simulink model "Ejercicio_2"  (R2020a)
settings: Solver=ode3  StartTime=0.0  StopTime=100.0  FixedStep=0.01  RelTol=1e-3
undefined symbols (not defined in the file or in its folder): DiscIntNeverNeededParam
libraries: simulink x1
settings Model: EnablePacing=on  Creator=atien  LastModifiedBy=atien

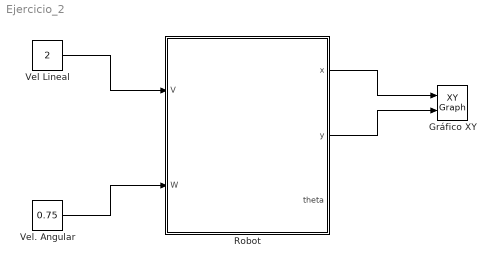
== system Ejercicio_2 ==
  Gráfico XY : simulink/Sinks/XY Graph  xmin=-10  xmax=10  ymin=-10  ymax=10  st=-1
  Robot : Subsystem
  Vel Lineal : Constant  Value=2
  Vel. Angular : Constant  Value=0.75
  wires:
  Vel Lineal/1 -> Robot/1(V)
  Robot/1(x) -> Gráfico XY/1
  Robot/2(y) -> Gráfico XY/2
  Vel. Angular/1 -> Robot/2(W)

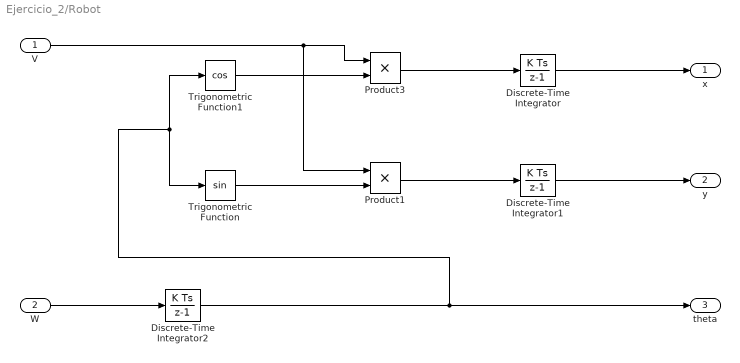
== system Ejercicio_2/Robot ==
  V : Inport
  W : Inport  Port=2
  Discrete-Time Integrator : DiscreteIntegrator  InitialCondition=-4  SampleTime=-1  ICPrevOutput=DiscIntNeverNeededParam  ICPrevScaledInput=DiscIntNeverNeededParam
  Discrete-Time Integrator1 : DiscreteIntegrator  InitialCondition=-4  SampleTime=-1  ICPrevOutput=DiscIntNeverNeededParam  ICPrevScaledInput=DiscIntNeverNeededParam
  Discrete-Time Integrator2 : DiscreteIntegrator  SampleTime=-1  ICPrevOutput=DiscIntNeverNeededParam  ICPrevScaledInput=DiscIntNeverNeededParam
  Product1 : Product
  Product3 : Product
  Trigonometric Function : Trigonometry
  Trigonometric Function1 : Trigonometry  Operator=cos
  x : Outport
  y : Outport  Port=2
  theta : Outport  Port=3
  wires:
  V/1 -> Product1/1, Product3/1
  Product3/1 -> Discrete-Time Integrator/1
  W/1 -> Discrete-Time Integrator2/1
  Product1/1 -> Discrete-Time Integrator1/1
  Discrete-Time Integrator2/1 -> theta/1, Trigonometric Function/1, Trigonometric Function1/1
  Discrete-Time Integrator/1 -> x/1
  Trigonometric Function1/1 -> Product3/2
  Trigonometric Function/1 -> Product1/2
  Discrete-Time Integrator1/1 -> y/1
